simulink model "sampleModel1755"  (R2023a)
settings: Solver=VariableStepAuto  StartTime=0.0  StopTime=10.0  RelTol=1e-3
libraries: hdlsllib x3, simulink x1
settings Model: Creator=user1  LastModifiedBy=user1

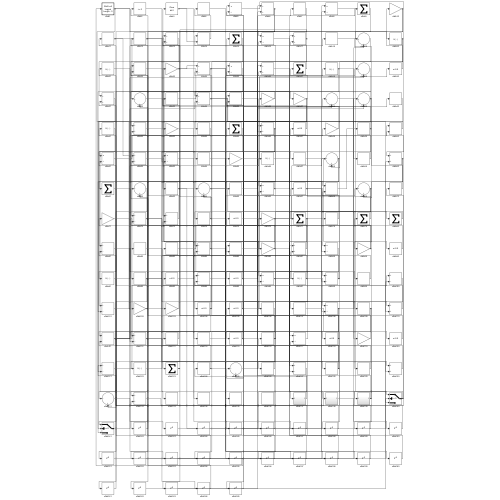
[thumbnail: Simulink's stored preview of the top-level diagram]
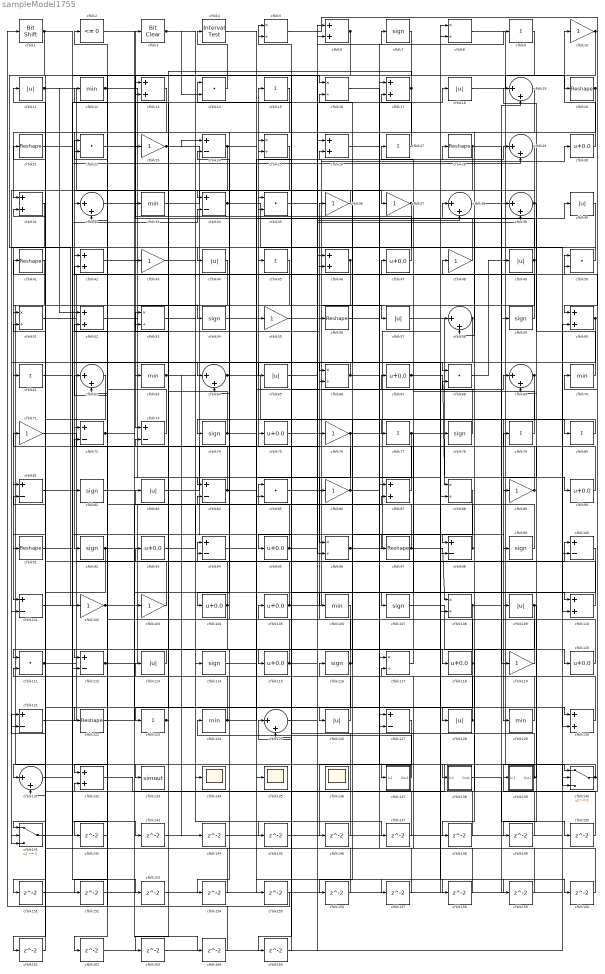
== system sampleModel1755 ==
  cfblk1 : hdlsllib/Logic and Bit Operations/Bit Shift  mode=Shift Left Logical  N=0
  cfblk{10,23,36..37,43,48,55,71,76,86,89,102..103,119} (14 alike) : Gain
  cfblk{24,34,72..73,81,84,94,98,100..101,112,121,127} (13 alike) : Sum  Inputs=+-
  cfblk{30,47,67,75,90,93,95,104..105,115,118,120} (12 alike) : Bias  Bias=0.0  SaturateOnIntegerOverflow=off
  cfblk{12,33,63,70,106,124,129} (7 alike) : MinMax
  cfblk{7,54,59,74,78,82,92,99,107,114,116} (11 alike) : Signum
  cfblk{5,8,16,25,51,53,66,88,96,108,117} (11 alike) : Product  Inputs=*/  RndMeth=Zero  SaturateOnIntegerOverflow=on
  cfblk{11,18,40,44,49,57,65,83,109,113,126,128} (12 alike) : Abs  SaturateOnIntegerOverflow=off
  cfblk{6,13,17,26,31,42,46,52,60,87,110,130,132} (13 alike) : Sum
  cfblk{14,22,35,50,68,85,111} (7 alike) : DotProduct  OutDataTypeStr=Inherit: Inherit via internal rule
  cfblk{20..21,28,41,56,91,97,122} (8 alike) : Reshape
  cfblk{9,15,27,45,61,77,79..80,123} (9 alike) : Sum  Inputs=+
  cfblk{19,29,32,38..39,58,62,64,69,125,131} (11 alike) : Sum  Inputs=|++
  cfblk133 : ToWorkspace  VariableName=simout  SaveFormat=Timeseries  SampleTime=-1
  cfblk134 : Scope
  cfblk135 : Scope
  cfblk136 : Scope
      settings: Floating=on
  cfblk137 : Subsystem
      settings: LibrarySourceBlock=|
      | hdlsllib/Ports &
      | Subsystems/Subsystem
  cfblk138 : Subsystem
      settings: LibrarySourceBlock=|
      | hdlsllib/Ports &
      | Subsystems/Subsystem
  cfblk139 : Subsystem
      settings: LibrarySourceBlock=|
      | hdlsllib/Ports &
      | Subsystems/Subsystem
  cfblk140 : Switch  SaturateOnIntegerOverflow=off  InputSameDT=off
  cfblk141 : Switch  SaturateOnIntegerOverflow=off  InputSameDT=off
  cfblk{142..165} (24 alike) : Delay  SampleTime=1
  cfblk2 : hdlsllib/Logic and Bit Operations/Compare To Zero  relop=<=  OutDataTypeStr=boolean
  cfblk3 : simulink/Logic and Bit Operations/Bit Clear  iBit=0
      settings: LibrarySourceBlock=|
      | hdlsllib/Logic and Bit
      | Operations/Bit Clear
  cfblk4 : hdlsllib/Logic and Bit Operations/Interval Test  IntervalClosedRight=on  uplimit=0.5  IntervalClosedLeft=on  lowlimit=-0.5  OutDataTypeStr=boolean
  wires:
  cfblk86/1 -> cfblk15/1, cfblk110/1
  cfblk8/1 -> cfblk140/1
  cfblk96/1 -> cfblk69/1, cfblk138/1(In1)
  cfblk111/1 -> cfblk45/1, cfblk56/1, cfblk50/1, cfblk34/2
  cfblk83/1 -> cfblk75/1
  cfblk24/1 -> cfblk43/1, cfblk157/1, cfblk158/1
  cfblk57/1 -> cfblk90/1
  cfblk41/1 -> cfblk133/1
  cfblk34/1 -> cfblk117/1, cfblk110/2
  cfblk33/1 -> cfblk37/1
  cfblk105/1 -> cfblk30/1, cfblk21/1
  cfblk104/1 -> cfblk94/1, cfblk24/2, cfblk161/1
  cfblk137/1(Out1) -> cfblk124/1
  cfblk30/1 -> cfblk10/1
  cfblk13/1 -> cfblk31/1
  cfblk79/1 -> cfblk27/1
  cfblk99/1 -> cfblk83/1
  cfblk68/1 -> cfblk49/1
  cfblk67/1 -> cfblk88/1, cfblk80/1
  cfblk121/1 -> cfblk100/1
  cfblk17/1 -> cfblk92/1, cfblk122/1
  cfblk119/1 -> cfblk105/1
  cfblk1/1 -> cfblk102/1, cfblk16/1, cfblk98/2
  cfblk132/1 -> cfblk70/1
  cfblk51/1 -> cfblk48/1
  cfblk44/1 -> cfblk101/1
  cfblk112/1 -> cfblk55/1, cfblk130/2
  cfblk31/1 -> cfblk81/1
  cfblk23/1 -> cfblk135/1, cfblk24/1
  cfblk63/1 -> cfblk144/1, cfblk145/1
  cfblk18/1 -> cfblk20/1
  cfblk14/1 -> cfblk4/1
  cfblk110/1 -> cfblk94/2
  cfblk64/1 -> cfblk129/1, cfblk86/1
  cfblk5/1 -> cfblk60/1
  cfblk75/1 -> cfblk29/1
  cfblk52/1 -> cfblk84/1
  cfblk58/1 -> cfblk95/1, cfblk162/1
  cfblk113/1 -> cfblk112/1
  cfblk42/1 -> cfblk114/1
  cfblk26/1 -> cfblk128/1
  cfblk90/1 -> cfblk11/1
  cfblk120/1 -> cfblk36/1
  cfblk19/1 -> cfblk72/1
  cfblk84/1 -> cfblk53/1, cfblk147/1
  cfblk49/1 -> cfblk3/1, cfblk64/1
  cfblk20/1 -> cfblk58/2, cfblk46/2
  cfblk55/1 -> cfblk57/1
  cfblk6/1 -> cfblk132/1, cfblk96/2
  cfblk130/1 -> cfblk41/1
  cfblk141/1 -> cfblk82/1
  cfblk32/1 -> cfblk96/1
  cfblk60/1 -> cfblk121/2, cfblk69/2
  cfblk102/1 -> cfblk2/1, cfblk130/1
  cfblk12/1 -> cfblk54/1, cfblk164/1
  cfblk82/1 -> cfblk106/1
  cfblk39/1 -> cfblk32/1, cfblk89/1, cfblk141/3
  cfblk76/1 -> cfblk8/2, cfblk85/2, cfblk140/3
  cfblk128/1 -> cfblk116/1, cfblk52/2
  cfblk74/1 -> cfblk40/1, cfblk13/2
  cfblk107/1 -> cfblk120/1
  cfblk48/1 -> cfblk5/1
  cfblk81/1 -> cfblk112/2
  cfblk77/1 -> cfblk107/1, cfblk127/2, cfblk160/1
  cfblk129/1 -> cfblk85/1
  cfblk11/1 -> cfblk127/1, cfblk52/1
  cfblk45/1 -> cfblk51/1
  cfblk115/1 -> cfblk28/1, cfblk33/1
  cfblk109/1 -> cfblk148/1, cfblk149/1
  cfblk85/1 -> cfblk67/1
  cfblk103/1 -> cfblk93/1
  cfblk124/1 -> cfblk71/1, cfblk66/2
  cfblk69/1 -> cfblk74/1, cfblk126/1
  cfblk100/1 -> cfblk125/2
  cfblk71/1 -> cfblk76/1
  cfblk37/1 -> cfblk73/1, cfblk101/2
  cfblk117/1 -> cfblk47/1
  cfblk116/1 -> cfblk16/2, cfblk64/2, cfblk142/1
  cfblk43/1 -> cfblk134/1
  cfblk10/1 -> cfblk123/1, cfblk141/1
  cfblk125/1 -> cfblk6/2
  cfblk28/1 -> cfblk119/1, cfblk141/2
  cfblk101/1 -> cfblk29/2
  cfblk3/1 -> cfblk97/1, cfblk14/2
  cfblk140/1 -> cfblk139/1(In1), cfblk50/2
  cfblk89/1 -> cfblk32/2, cfblk25/2
  cfblk59/1 -> cfblk22/1
  cfblk122/1 -> cfblk84/2
  cfblk108/1 -> cfblk39/1, cfblk131/2, cfblk154/1
  cfblk87/1 -> cfblk62/2
  cfblk9/1 -> cfblk63/1
  cfblk118/1 -> cfblk22/2, cfblk131/1, cfblk13/1
  cfblk15/1 -> cfblk104/1
  cfblk21/1 -> cfblk65/1
  cfblk56/1 -> cfblk99/1
  cfblk53/1 -> cfblk109/1
  cfblk97/1 -> cfblk108/1, cfblk35/1
  cfblk50/1 -> cfblk42/1
  cfblk62/1 -> cfblk91/1
  cfblk36/1 -> cfblk34/1
  cfblk95/1 -> cfblk42/2, cfblk39/2
  cfblk2/1 -> cfblk137/1(In1)
  cfblk27/1 -> cfblk17/2
  cfblk78/1 -> cfblk25/1
  cfblk54/1 -> cfblk108/2
  cfblk123/1 -> cfblk73/2, cfblk163/1
  cfblk29/1 -> cfblk66/1
  cfblk73/1 -> cfblk12/1
  cfblk70/1 -> cfblk19/1
  cfblk66/1 -> cfblk61/1, cfblk9/1
  cfblk93/1 -> cfblk87/2
  cfblk16/1 -> cfblk68/1
  cfblk98/1 -> cfblk38/1, cfblk35/2
  cfblk40/1 -> cfblk44/1
  cfblk139/1(Out1) -> cfblk79/1, cfblk14/1
  cfblk46/1 -> cfblk115/1, cfblk53/2
  cfblk72/1 -> cfblk103/1, cfblk88/2
  cfblk35/1 -> cfblk38/2
  cfblk91/1 -> cfblk18/1
  cfblk114/1 -> cfblk26/2
  cfblk92/1 -> cfblk111/1, cfblk118/1, cfblk98/1
  cfblk126/1 -> cfblk113/1
  cfblk38/1 -> cfblk59/1
  cfblk22/1 -> cfblk78/1
  cfblk47/1 -> cfblk23/1
  cfblk80/1 -> cfblk77/1
  cfblk65/1 -> cfblk7/1
  cfblk142/1 -> cfblk62/1
  cfblk61/1 -> cfblk143/1
  cfblk143/1 -> cfblk26/1
  cfblk144/1 -> cfblk58/1
  cfblk145/1 -> cfblk60/2
  cfblk127/1 -> cfblk146/1
  cfblk146/1 -> cfblk6/1
  cfblk147/1 -> cfblk81/2
  cfblk148/1 -> cfblk31/2
  cfblk149/1 -> cfblk68/2
  cfblk138/1(Out1) -> cfblk150/1
  cfblk150/1 -> cfblk121/1
  cfblk25/1 -> cfblk151/1
  cfblk151/1 -> cfblk19/2
  cfblk106/1 -> cfblk152/1
  cfblk152/1 -> cfblk140/2
  cfblk131/1 -> cfblk153/1
  cfblk153/1 -> cfblk8/1
  cfblk154/1 -> cfblk51/2
  cfblk4/1 -> cfblk155/1
  cfblk155/1 -> cfblk1/1
  cfblk88/1 -> cfblk156/1
  cfblk156/1 -> cfblk5/2
  cfblk157/1 -> cfblk87/1
  cfblk158/1 -> cfblk117/2
  cfblk94/1 -> cfblk159/1
  cfblk159/1 -> cfblk17/1
  cfblk160/1 -> cfblk72/2
  cfblk161/1 -> cfblk111/2
  cfblk162/1 -> cfblk100/2
  cfblk163/1 -> cfblk46/1
  cfblk164/1 -> cfblk132/2
  cfblk7/1 -> cfblk165/1
  cfblk165/1 -> cfblk125/1

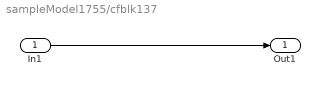
== system sampleModel1755/cfblk137 ==
  In1 : Inport
  Out1 : Outport
  wires:
  In1/1 -> Out1/1

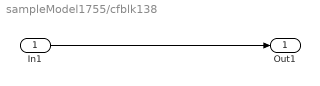
== system sampleModel1755/cfblk138 ==
  In1 : Inport
  Out1 : Outport
  wires:
  In1/1 -> Out1/1

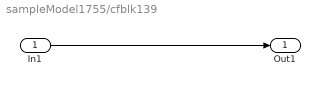
== system sampleModel1755/cfblk139 ==
  In1 : Inport
  Out1 : Outport
  wires:
  In1/1 -> Out1/1
